simulink library "pm_engine"  (Simulink 6.0)
settings: Solver=ode45  SolverMode=SingleTasking  StartTime=0.0  StopTime=10.0  RelTol=1e-3
undefined symbols (not defined in the file or in its folder): gcbh, mech_set_param
libraries: pm_engine x2
settings Model: Creator=nbrewton  LastModifiedBy=batserve  ExtModeAutoUpdateStatusClock=off
settings DataIOCC: SignalLoggingName=logsOut
settings OptimizationCC: BooleanDataType=off
settings DebuggingCC: CheckExecutionContextPreStartOutputMsg=on  CheckExecutionContextRuntimeOutputMsg=on  SolverPrmCheckMsg=none
settings HardwareCC: TargetUnknown=on

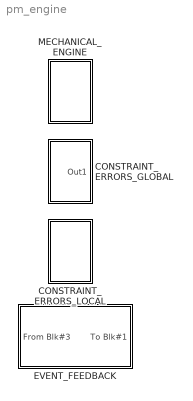
== system pm_engine ==
  CONSTRAINT_ERRORS_GLOBAL : Subsystem  InitFcn=mech_set_param(gcbh,'Tags','');  mask{Tags=}
      mask init:
      | mech_constraintOutput('maskinitglobal', gcbh, Tags);
  CONSTRAINT_ERRORS_LOCAL : Subsystem  mask(ConstraintErrorBlock){GotoTag=A, NumInputs=0}
      mask prompts: GotoTag "Goto Tag"; NumInputs "Num Inputs"
      mask init:
      | mech_constraintOutput('maskinitlocal', gcbh, GotoTag, NumInputs);
  EVENT_FEEDBACK : Subsystem  mask(Event Feedback){ic=2, k=0.5, x=1.0, ModeIteration=1}
      mask prompts: ic "InitialCondition"; k "Gain"; x "Constant"
      mask init:
      | sfun = [getfullname(gcbh) '/sfun_event_feedback'];
      | set_param(sfun, 'Parameters', ...
      | 	num2str(feature('SimMechanicsModeIteration')));
  MECHANICAL_ENGINE : Subsystem  mask{MachineId=0}
      mask init:
      | mech_initGround('engine', gcbh, MachineId);

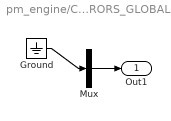
== system pm_engine/CONSTRAINT_ERRORS_GLOBAL ==
  Ground : Ground
  Mux : Mux  Inputs=1
  Out1 : Outport
  wires:
  Mux/1 -> Out1/1
  Ground/1 -> Mux/1

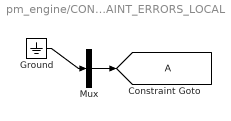
== system pm_engine/CONSTRAINT_ERRORS_LOCAL ==
  Ground : Ground
  Mux : Mux  Inputs=1
  tag scope: A=global
  wires:
  Mux/1 -> [A]
  Ground/1 -> Mux/1

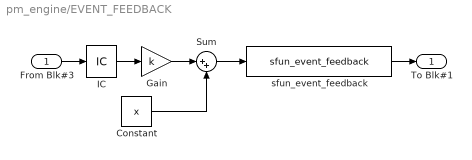
== system pm_engine/EVENT_FEEDBACK ==
  From Blk#3 : Inport  Port=1  LatchInput=off
  Constant : Constant  Value=x
  Gain : Gain  Gain=k  SaturateOnIntegerOverflow=on
  IC : InitialCondition  Value=ic
  Sum : Sum  Inputs=|++  SaturateOnIntegerOverflow=on  InputSameDT=on
  sfun_event_feedback : S-Function  FunctionName=sfun_event_feedback  Parameters=1
  To Blk#1 : Outport
  wires:
  Gain/1 -> Sum/1
  IC/1 -> Gain/1
  Constant/1 -> Sum/2
  From Blk#3/1 -> IC/1
  Sum/1 -> sfun_event_feedback/1
  sfun_event_feedback/1 -> To Blk#1/1

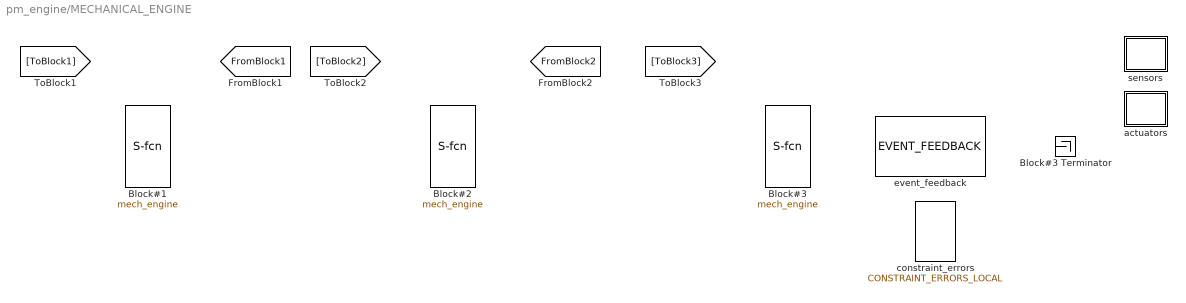
== system pm_engine/MECHANICAL_ENGINE ==
  Block#1 : S-Function  FunctionName=mech_engine  Parameters=1,0
  Block#2 : S-Function  FunctionName=mech_engine  Parameters=2,0
  Block#3 : S-Function  FunctionName=mech_engine  Parameters=3,0
  Block#3 Terminator : Terminator
  actuators : Subsystem
  constraint_errors : pm_engine/CONSTRAINT_ERRORS_LOCAL  GotoTag=A  NumInputs=0
  event_feedback : pm_engine/EVENT_FEEDBACK  ic=2  k=0.5  x=1.0  ModeIteration=1
  sensors : Subsystem
  tag scope: FromBlock1=global, FromBlock2=global

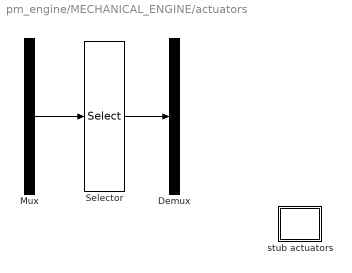
== system pm_engine/MECHANICAL_ENGINE/actuators ==
  Demux : Demux  Outputs=3
  Mux : Mux  Inputs=3
  Selector : Selector  Elements=[1 2 3]  InputPortWidth=3
  stub actuators : Subsystem
  wires:
  Selector/1 -> Demux/1
  Mux/1 -> Selector/1

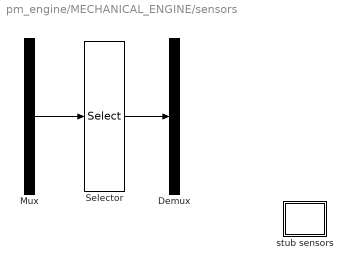
== system pm_engine/MECHANICAL_ENGINE/sensors ==
  Demux : Demux  Outputs=2
  Mux : Mux  Inputs=2
  Selector : Selector  Elements=[1 2]  InputPortWidth=2
  stub sensors : Subsystem
  wires:
  Selector/1 -> Demux/1
  Mux/1 -> Selector/1

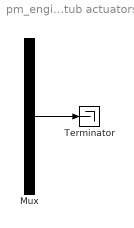
== system pm_engine/MECHANICAL_ENGINE/actuators/stub actuators ==
  Mux : Mux  Inputs=2
  Terminator : Terminator
  wires:
  Mux/1 -> Terminator/1

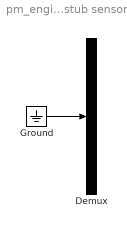
== system pm_engine/MECHANICAL_ENGINE/sensors/stub sensors ==
  Demux : Demux  Outputs=2
  Ground : Ground
  wires:
  Ground/1 -> Demux/1
